simulink model "Prob_9"  (R2020b)
settings: Solver=VariableStepAuto  StartTime=0.0  StopTime=10.0  RelTol=1e-3
model workspace (MAT data in the model file):
  J = 0.05
  K = 0.01
  L = 0.5
  R = 1
  b = 0.1
settings Model: Creator=Lakshmi  LastModifiedBy=Lakshmi

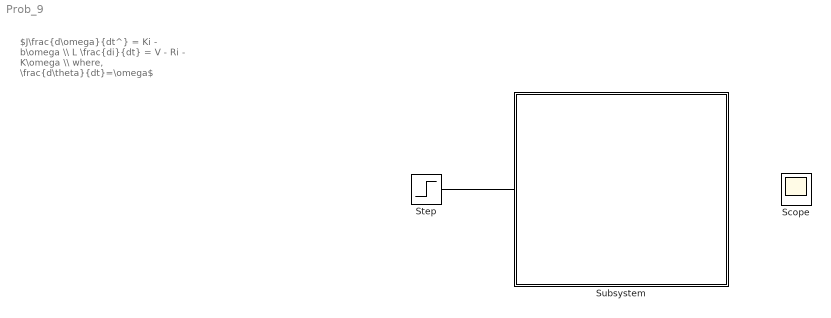
== system Prob_9 ==
  note: $J\frac{d\omega}{dt^} = Ki - b\omega \\ L \frac{di}{dt} = V - Ri - K\omega \\ where, \frac{d\theta}{dt}=\omega$
  Scope : Scope
  Step : Step  SampleTime=0
  Subsystem : Subsystem
  wires:
  Step/1 -> ?
  ? -> Scope/1

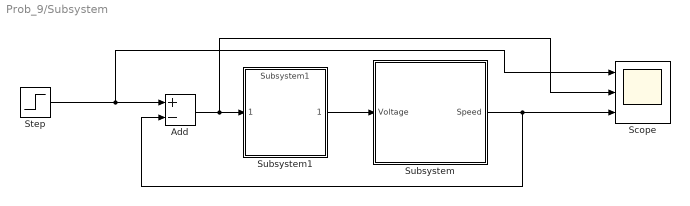
== system Prob_9/Subsystem ==
  Add : Sum  Inputs=+-
  Scope : Scope  NumInputPorts=3
  Step : Step  After=4  SampleTime=0
  Subsystem : Subsystem
  Subsystem1 : ModelReference  ModelNameDialog=Subsystem1  SimulationMode=Normal  ModelReferenceVersion=1.5
  wires:
  Subsystem/1(Speed) -> Add/2, Scope/3
  Step/1 -> Scope/1, Add/1
  Add/1 -> Subsystem1/1, Scope/2
  Subsystem1/1 -> Subsystem/1(Voltage)

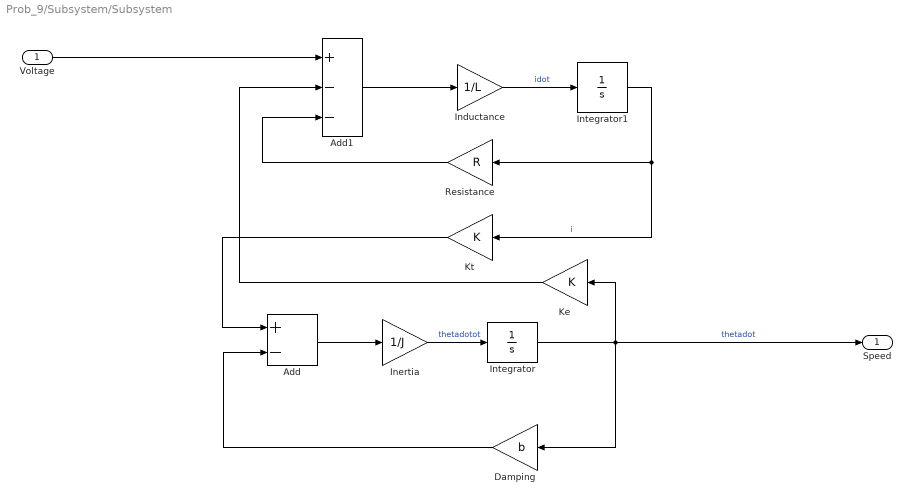
== system Prob_9/Subsystem/Subsystem ==
  Voltage : Inport
  Add : Sum  Inputs=+-
  Add1 : Sum  Inputs=+--
  Damping : Gain  Gain=b
  Inductance : Gain  Gain=1/L
  Inertia : Gain  Gain=1/J
  Integrator : Integrator
  Integrator1 : Integrator
  Ke : Gain  Gain=K
  Kt : Gain  Gain=K
  Resistance : Gain  Gain=R
  Speed : Outport
  wires:
  Add1/1 -> Inductance/1
  Resistance/1 -> Add1/3
  Integrator/1 -> Speed/1, Ke/1, Damping/1  "thetadot"
  Inertia/1 -> Integrator/1  "thetadotot"
  Add/1 -> Inertia/1
  Inductance/1 -> Integrator1/1  "idot"
  Damping/1 -> Add/2
  Kt/1 -> Add/1
  Integrator1/1 -> Kt/1, Resistance/1  "i"
  Ke/1 -> Add1/2
  Voltage/1 -> Add1/1
